simulink model "continuousDynamics"  (R2018b)
settings: Solver=VariableStepAuto  StartTime=0.0  StopTime=10.0  RelTol=1e-3
settings Model: Creator=feiyang  LastModifiedBy=feiyang

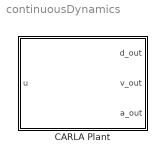
== system continuousDynamics ==
  CARLA Plant : Stateflow chart  TreatAsAtomicUnit=on

== stateflow chart continuousDynamics/CARLA Plant ==
  settings: updateMethod=CONTINUOUS
  state Brake
    du:
    d_dot = v;
    v_dot = u;
    d_out = d;
    v_out = v;
    a_out = u;
  (default) -> Brake : {d=0;
      | v=0;}
  data: d local; v local; u input; d_out output; v_out output; a_out output
